simulink model "ActiveControl"  (R2023a)
settings: Solver=FixedStepAuto  StartTime=0.0  StopTime=inf  RelTol=1e-3
libraries: ros2lib x4

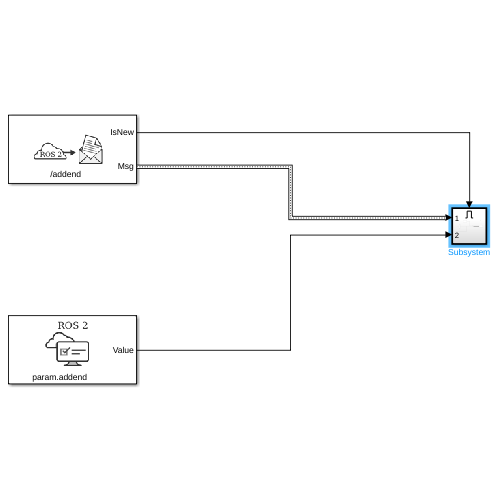
[thumbnail: Simulink's stored preview of the top-level diagram]
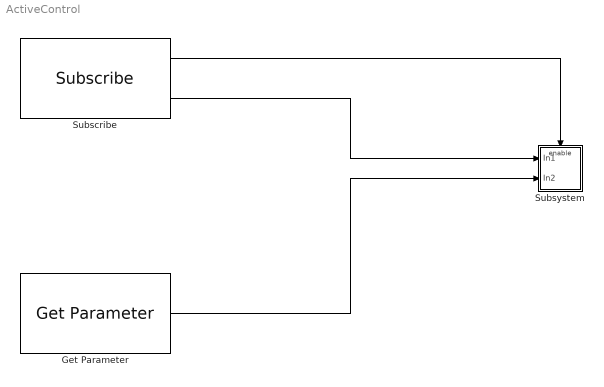
== system ActiveControl ==
  Get Parameter : ros2lib/Get Parameter  ParameterName=param.addend  ParameterType=int64  ParameterMaxArrayLength=16  ParameterInitialValue=0  SampleTime=-1  ModelName=ActiveControl  BlockId=ParamGet_ActiveControl_3
  Subscribe : ros2lib/Subscribe  topicSource=Specify your own  topic=/addend  messageType=std_msgs/Int64  sampleTime=-1  QOSHistory=Keep last  QOSDepth=1  QOSReliability=Reliable  QOSDurability=Volatile
  Subsystem : Subsystem
  wires:
  Subscribe/2 -> Subsystem/1(In1)
  Get Parameter/1 -> Subsystem/2(In2)
  Subscribe/1 -> Subsystem/Enable

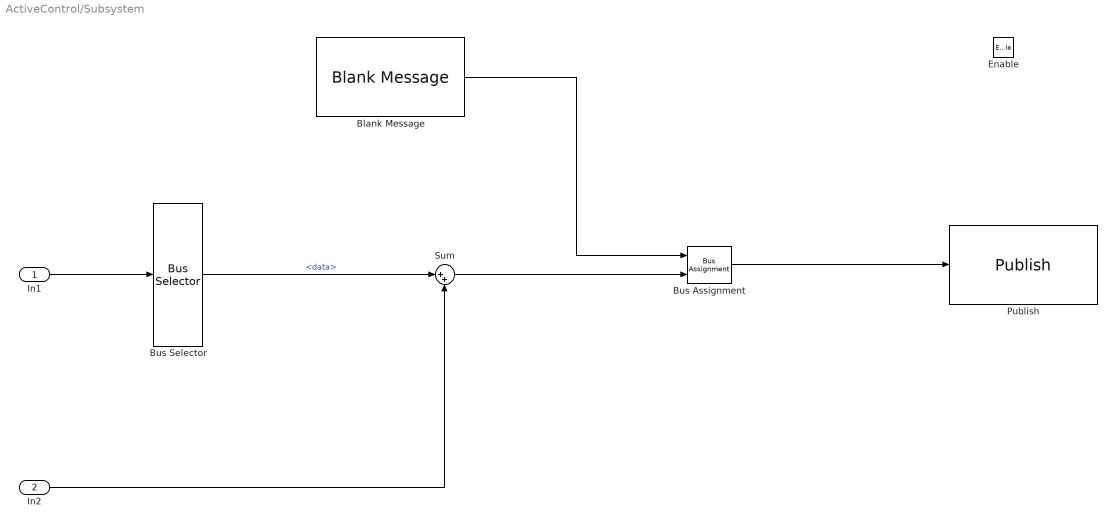
== system ActiveControl/Subsystem ==
  In1 : Inport
  In2 : Inport  Port=2
  Enable : EnablePort
  Blank Message : ros2lib/Blank Message  messageClass=Message  entityType=std_msgs/Int64  messageType=std_msgs/Int64  SampleTime=-1
  Bus Assignment : BusAssignment  AssignedSignals=data
  Bus Selector : BusSelector  OutputSignals=data
  Publish : ros2lib/Publish  topicSource=Specify your own  topic=/sum  messageType=std_msgs/Int64  QOSHistory=Keep last  QOSDepth=1  QOSReliability=Reliable  QOSDurability=Volatile
  Sum : Sum  Inputs=|++
  wires:
  Sum/1 -> Bus Assignment/2
  Blank Message/1 -> Bus Assignment/1
  Bus Selector/1 -> Sum/1  "<data>"
  Bus Assignment/1 -> Publish/1
  In1/1 -> Bus Selector/1
  In2/1 -> Sum/2
